simulink library "DYN_EPHEM"  (Simulink 8.8)
settings: Solver=ode45  StartTime=0.0  StopTime=10.0  RelTol=1e-3  EnableMultiTasking=on
libraries: LIB_ROT x4
settings Model: Creator=alger  LastModifiedBy=alger

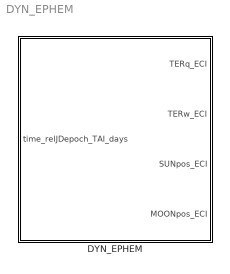
== system DYN_EPHEM ==
  DYN_EPHEM : Subsystem

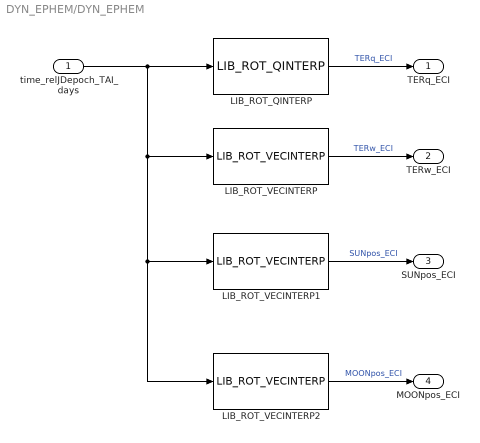
== system DYN_EPHEM/DYN_EPHEM ==
  time_relJDepoch_TAI_days : Inport  PortDimensions=1
  LIB_ROT_QINTERP : LIB_ROT/LIB_ROT_QINTERP  time_start=EARTHstates.time_relJDepoch_TAI_days_start  time_step=EARTHstates.time_relJDepoch_TAI_days_step  Bq_A_ref=EARTHstates.BCBFq_CEL
  LIB_ROT_VECINTERP : LIB_ROT/LIB_ROT_VECINTERP  time_start=EARTHstates.time_relJDepoch_TAI_days_start  time_step=EARTHstates.time_relJDepoch_TAI_days_step  vec_ref=EARTHstates.BCBFw_relCEL_BCBF
  LIB_ROT_VECINTERP1 : LIB_ROT/LIB_ROT_VECINTERP  time_start=SUNstates.time_relJDepoch_TAI_days_start  time_step=SUNstates.time_relJDepoch_TAI_days_step  vec_ref=SUNstates.BODYpos_ref
  LIB_ROT_VECINTERP2 : LIB_ROT/LIB_ROT_VECINTERP  time_start=MOONstates.time_relJDepoch_TAI_days_start  time_step=MOONstates.time_relJDepoch_TAI_days_step  vec_ref=MOONstates.BODYpos_ref
  TERq_ECI : Outport  PortDimensions=4
  TERw_ECI : Outport  Port=2  PortDimensions=3
  SUNpos_ECI : Outport  Port=3  PortDimensions=3
  MOONpos_ECI : Outport  Port=4  PortDimensions=3
  wires:
  LIB_ROT_QINTERP/1 -> TERq_ECI/1  "TERq_ECI"
  LIB_ROT_VECINTERP/1 -> TERw_ECI/1  "TERw_ECI"
  time_relJDepoch_TAI_days/1 -> LIB_ROT_VECINTERP2/1, LIB_ROT_VECINTERP1/1, LIB_ROT_VECINTERP/1, LIB_ROT_QINTERP/1
  LIB_ROT_VECINTERP1/1 -> SUNpos_ECI/1  "SUNpos_ECI"
  LIB_ROT_VECINTERP2/1 -> MOONpos_ECI/1  "MOONpos_ECI"
